simulink model "QuaterCar_Model"  (R2018b)
settings: Solver=VariableStepAuto  StartTime=0.0  StopTime=10  RelTol=1e-10
values from neighbouring files (symbols this model uses):
  csc = 600    [SetCoefficients.m]    (also in SetCoefficients_HC.m)
  cse = 1200    [SetCoefficients.m]    (also in SetCoefficients_HC.m)
  g = 9.81    [SetCoefficients.m]    (also in SetCoefficients_HC.m)
  ks = 2e4    (= 20000)    [SetCoefficients.m]    (also in SetCoefficients_HC.m)
  ksstiff = 20*ks    (= 400000)    [SetCoefficients.m]    (also in SetCoefficients_HC.m)
  kt = 14e4    (= 140000)    [SetCoefficients.m]    (also in SetCoefficients_HC.m)
  m1 = mb/2    (= 250)    [SetCoefficients.m]    (also in SetCoefficients_HC.m)
  m2 = 20    [SetCoefficients.m]    (also in SetCoefficients_HC.m)
  x1 = 0.2    [SetCoefficients.m]    (also in SetCoefficients_HC.m)
  x2 = 0.5    [SetCoefficients.m]    (also in SetCoefficients_HC.m)
settings Model: Creator=joebe  LastModifiedBy=joebe
settings SolverCC: ZeroCrossAlgorithm=Adaptive
settings DebuggingCC: IgnoredZcDiagnostic=none

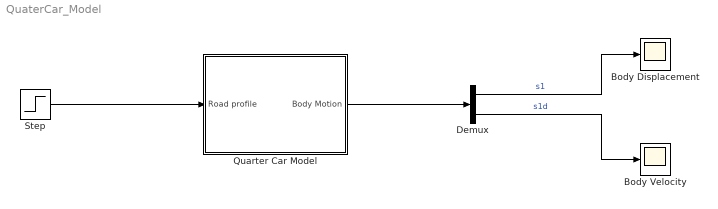
== system QuaterCar_Model ==
  Body Displacement : Scope
  Body Velocity : Scope
  Demux : Demux  Outputs=2
  Quarter Car Model : Subsystem
  Step : Step  Time=3  After=.1  SampleTime=0
  wires:
  Demux/1 -> Body Displacement/1  "s1"
  Demux/2 -> Body Velocity/1  "s1d"
  Quarter Car Model/1(Body Motion) -> Demux/1
  Step/1 -> Quarter Car Model/1(Road profile)

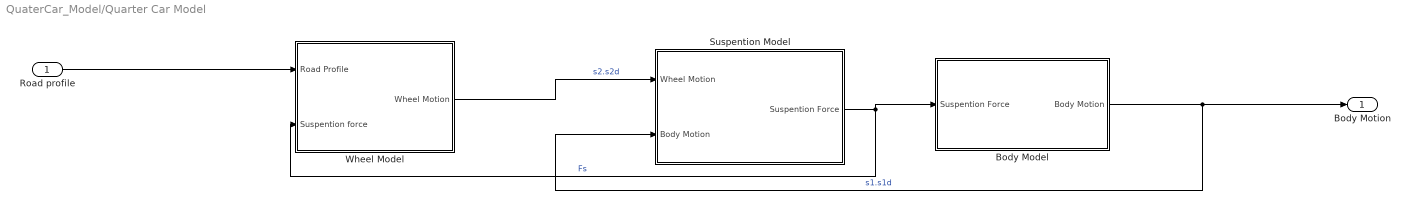
== system QuaterCar_Model/Quarter Car Model ==
  Road profile : Inport
  Body Model : Subsystem
  Suspention Model : Subsystem
  Wheel Model : Subsystem
  Body Motion : Outport
  wires:
  Suspention Model/1(Suspention Force) -> Body Model/1("Suspention Force "), Wheel Model/2(Suspention force)  "Fs"
  Wheel Model/1(Wheel Motion) -> Suspention Model/1(Wheel Motion)  "s2.s2d"
  Body Model/1(Body Motion) -> Suspention Model/2(Body Motion), Body Motion/1  "s1.s1d"
  Road profile/1 -> Wheel Model/1(Road Profile)

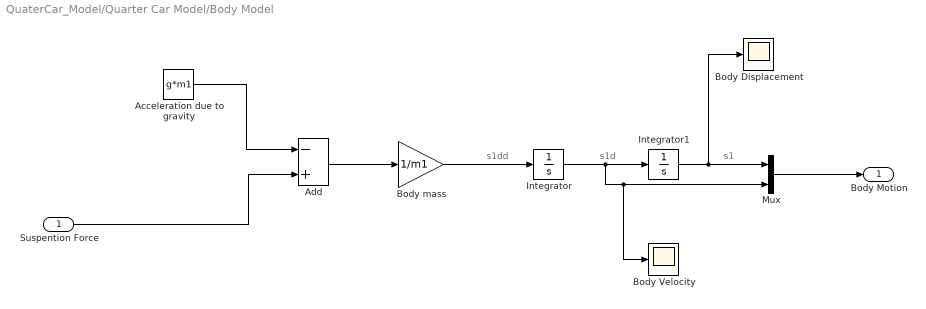
== system QuaterCar_Model/Quarter Car Model/Body Model ==
  note: s1d
  note: s1
  note: s1dd
  "Suspention Force " : Inport
  Acceleration due to gravity : Constant  Value=g*m1
  Add : Sum  Inputs=-+
  Body Displacement : Scope
  Body Velocity : Scope
  Body mass : Gain  Gain=1/m1
  Integrator : Integrator
  Integrator1 : Integrator
  Mux : Mux  Inputs=2
  Body Motion : Outport
  wires:
  "Suspention Force "/1 -> Add/2
  Integrator/1 -> Body Velocity/1, Mux/2, Integrator1/1
  Add/1 -> Body mass/1
  Acceleration due to gravity/1 -> Add/1
  Integrator1/1 -> Body Displacement/1, Mux/1
  Mux/1 -> Body Motion/1
  Body mass/1 -> Integrator/1

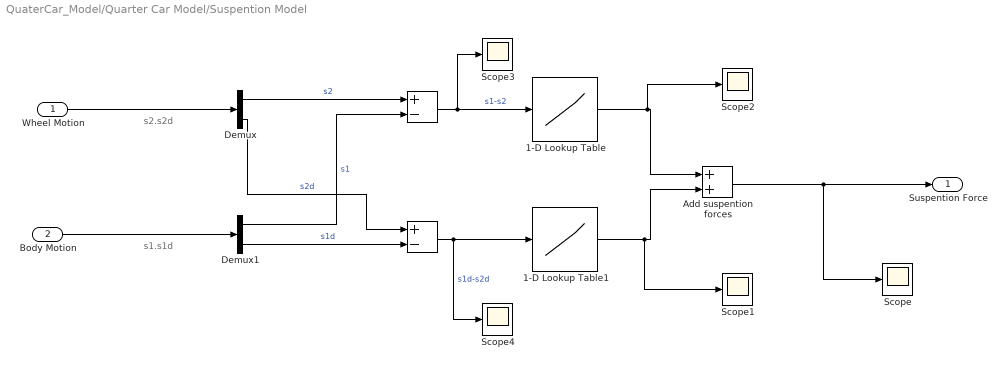
== system QuaterCar_Model/Quarter Car Model/Suspention Model ==
  note: s1.s1d
  note: s2.s2d
  Wheel Motion : Inport
  Body Motion : Inport  Port=2
  " " : Sum  Inputs=+-
  " " : Sum  Inputs=+-
  1-D Lookup Table : Lookup_n-D  NumberOfTableDimensions=1  BreakpointsForDimension1=[-x2 -x1 x1 x2]  Table=[-(ksstiff*(x2-x1)+ks*x1) -x1*ks x1*ks (ksstiff*(x2-x1)+ks*x1)]  InternalRulePriority=Speed  RndMeth=Simplest  InputSameDT=on
  1-D Lookup Table1 : Lookup_n-D  NumberOfTableDimensions=1  BreakpointsForDimension1=[-10 0 10]  Table=[-10*cse 0 10*csc]  InternalRulePriority=Speed  RndMeth=Simplest  InputSameDT=on
  Add suspention forces : Sum
  Demux : Demux  Outputs=2
  Demux1 : Demux  Outputs=2
  Scope{,1..4} (5 alike) : Scope
  Suspention Force : Outport
  wires:
  Demux1/2 -> " "/2  "s1d"
  " "/1 -> Scope3/1, 1-D Lookup Table/1  "s1-s2"
  Demux1/1 -> " "/2  "s1"
  1-D Lookup Table1/1 -> Scope1/1, Add suspention forces/2
  1-D Lookup Table/1 -> Scope2/1, Add suspention forces/1
  Demux/1 -> " "/1  "s2"
  Demux/2 -> " "/1  "s2d"
  Body Motion/1 -> Demux1/1
  " "/1 -> Scope4/1, 1-D Lookup Table1/1  "s1d-s2d"
  Add suspention forces/1 -> Scope/1, Suspention Force/1
  Wheel Motion/1 -> Demux/1

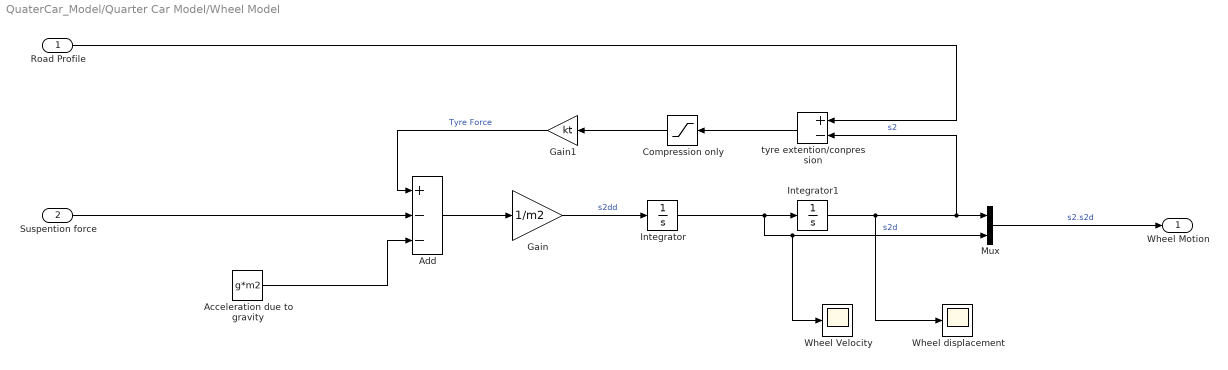
== system QuaterCar_Model/Quarter Car Model/Wheel Model ==
  Road Profile : Inport
  Suspention force : Inport  Port=2
  Acceleration due to gravity : Constant  Value=g*m2
  Add : Sum  Inputs=+--
  Compression only : Saturate  UpperLimit=inf  LowerLimit=0
  Gain : Gain  Gain=1/m2
  Gain1 : Gain  Gain=kt
  Integrator : Integrator
  Integrator1 : Integrator
  Mux : Mux  Inputs=2
  Wheel Velocity : Scope
  Wheel displacement : Scope
  tyre extention/conpression : Sum  Inputs=+-
  Wheel Motion : Outport
  wires:
  Integrator1/1 -> Wheel displacement/1, tyre extention/conpression/2, Mux/1  "s2"
  Integrator/1 -> Wheel Velocity/1, Mux/2, Integrator1/1  "s2d"
  Add/1 -> Gain/1
  Gain1/1 -> Add/1  "Tyre Force"
  Road Profile/1 -> tyre extention/conpression/1
  Mux/1 -> Wheel Motion/1  "s2.s2d"
  Acceleration due to gravity/1 -> Add/3
  Suspention force/1 -> Add/2
  Gain/1 -> Integrator/1  "s2dd"
  tyre extention/conpression/1 -> Compression only/1
  Compression only/1 -> Gain1/1
